simulink model "z2_symulacja"  (R2021a)
settings: Solver=VariableStepAuto  StartTime=0.0  StopTime=5  RelTol=1e-3
settings Model: Creator=48604  LastModifiedBy=48604

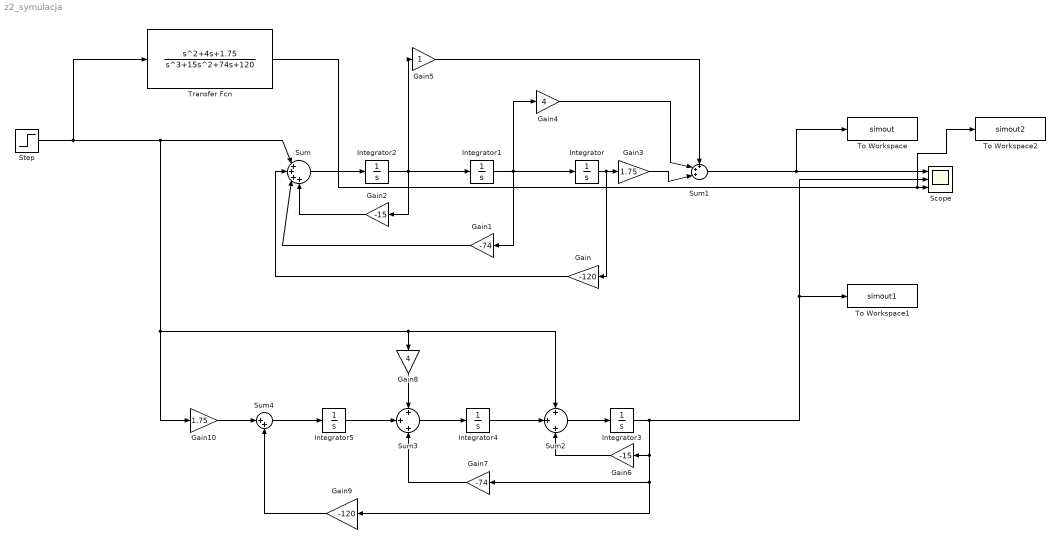
== system z2_symulacja ==
  Gain : Gain  Gain=-120
  Gain1 : Gain  Gain=-74
  Gain10 : Gain  Gain=1.75
  Gain2 : Gain  Gain=-15
  Gain3 : Gain  Gain=1.75
  Gain4 : Gain  Gain=4
  Gain5 : Gain
  Gain6 : Gain  Gain=-15
  Gain7 : Gain  Gain=-74
  Gain8 : Gain  Gain=4
  Gain9 : Gain  Gain=-120
  Integrator{,1..5} (6 alike) : Integrator
  Scope : Scope  NumInputPorts=3
  Step : Step  SampleTime=1
  Sum : Sum  Inputs=|++++
  Sum1 : Sum  Inputs=+++|
  Sum2 : Sum  Inputs=+|+|+
  Sum3 : Sum  Inputs=+|+|+
  Sum4 : Sum  Inputs=|++
  To Workspace : ToWorkspace  VariableName=simout  SaveFormat=Structure With Time  SampleTime=-1
  To Workspace1 : ToWorkspace  VariableName=simout1  SaveFormat=Structure With Time  SampleTime=-1
  To Workspace2 : ToWorkspace  VariableName=simout2  SaveFormat=Structure With Time  SampleTime=-1
  Transfer Fcn : TransferFcn  Numerator=[1 4 1.75]  Denominator=[1 15 74 120]
  wires:
  Integrator2/1 -> Integrator1/1, Gain2/1, Gain5/1
  Integrator1/1 -> Integrator/1, Gain1/1, Gain4/1
  Sum1/1 -> To Workspace/1, Scope/1
  Gain4/1 -> Sum1/2
  Gain/1 -> Sum/2
  Gain3/1 -> Sum1/3
  Gain5/1 -> Sum1/1
  Integrator/1 -> Gain/1, Gain3/1
  Gain1/1 -> Sum/3
  Sum/1 -> Integrator2/1
  Gain2/1 -> Sum/4
  Integrator3/1 -> To Workspace1/1, Scope/2, Gain9/1, Gain7/1, Gain6/1
  Gain6/1 -> Sum2/3
  Gain9/1 -> Sum4/2
  Gain10/1 -> Sum4/1
  Gain8/1 -> Sum3/1
  Integrator4/1 -> Sum2/2
  Step/1 -> Transfer Fcn/1, Gain10/1, Gain8/1, Sum2/1, Sum/1
  Sum2/1 -> Integrator3/1
  Sum3/1 -> Integrator4/1
  Integrator5/1 -> Sum3/2
  Gain7/1 -> Sum3/3
  Sum4/1 -> Integrator5/1
  Transfer Fcn/1 -> To Workspace2/1, Scope/3
